simulink model "tower_mpc"  (Simulink 7.9)
settings: Solver=VariableStepDiscrete  StartTime=0.0  StopTime=10.0  RelTol=1e-3
undefined symbols (not defined in the file or in its folder): tower, tower_x0, tower_xref, Ts
libraries: mpclib x1
settings Model: Creator=matias  LastModifiedBy=matias

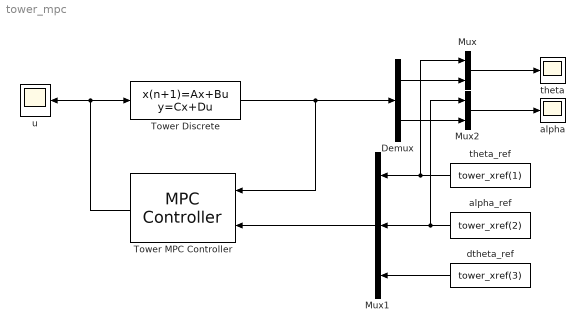
== system tower_mpc ==
  Demux : Demux  Outputs=2
  Mux : Mux  Inputs=2
  Mux1 : Mux  Inputs=3
  Mux2 : Mux  Inputs=2
  Tower Discrete : DiscreteStateSpace  A=tower.A  B=tower.B  C=tower.C(tower.OutputGroup.MO,:)  D=tower.D(tower.OutputGroup.MO,:)  X0=tower_x0  SampleTime=Ts
  Tower MPC Controller : mpclib/MPC Controller  mpcobj=tower_MPC  x0=[]  md_inport=off  mv_inport=off  lims_inport=off  switch_inport=off  ywt_inport=off  duwt_inport=off  rhoeps_inport=off  cost_outport=off  return_sequence=off  return_qpstatus=off  is_multiple=0  enable_value=0  n_mv=1  n_mo=2  n_md=0  n_ts=0.01  is_designfromscratch=0  ref_from_ws=off  ref_signal_name=[]  ref_preview=on  md_from_ws=off  md_signal_name=[]  md_preview=on  from_project=off  project_file=MPCtask.mat
  alpha : Scope
      settings: SaveName=ScopeData2
  alpha_ref : Constant  Value=tower_xref(2)
  dtheta_ref : Constant  Value=tower_xref(3)
  theta : Scope
  theta_ref : Constant  Value=tower_xref(1)
  u : Scope
  wires:
  Tower Discrete/1 -> Demux/1, Tower MPC Controller/1
  Tower MPC Controller/1 -> Tower Discrete/1, u/1
  Mux/1 -> theta/1
  theta_ref/1 -> Mux/1, Mux1/1
  Mux1/1 -> Tower MPC Controller/2
  Mux2/1 -> alpha/1
  Demux/1 -> Mux/2
  alpha_ref/1 -> Mux1/2, Mux2/1
  dtheta_ref/1 -> Mux1/3
  Demux/2 -> Mux2/2
